simulink library "tllib"  (R2015a)
settings: Solver=ode45  StartTime=0.0  StopTime=10.0  RelTol=1e-3
PostLoadFcn:
  | load_system('simulink')
libraries: simulink x6, tllib x3
(part 1 of 2)
CloseFcn:
  | if (bdIsLoaded('simulink')) && (strcmp(get_param('simulink', 'open'), 'off'))
  | close_system('simulink')
  | end;
settings Model: Creator=dSPACE GmbH  LastModifiedBy=dSPACE GmbH

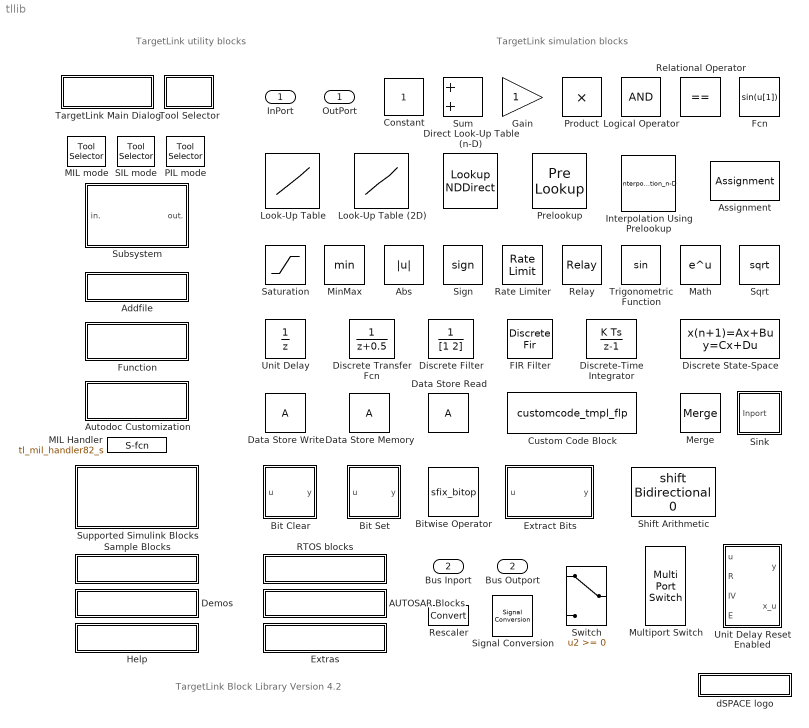
== system tllib ==
  note: TargetLink utility blocks
  note: TargetLink simulation blocks
  note: TargetLink Block Library Version 4.2
  InPort : Inport  mask(TL_Inport){data={'date',730486}}
      settings: CopyFcn=if exist('tl_copyfcntllib', 'file') == 2, tl_copyfcntllib(gcbh); end;  DeleteFcn=if exist('delete_tlblock','file')==2,delete_tlblock(gcbh);end  NameChangeFcn=if exist('rename_tlblock','file')==2,rename_tlblock(gcbh);end  OpenFcn=if exist('tl_open_blockdlg','file')==2,tl_open_blockdlg(gcbh);else,open_system(gcbh,'parameter');end
      mask Help: eval(['if exist(''tl_online_help'',''file'') == 2, tl_online_help(''Topic'',''TL_Inport''),else, web([''jar:file:///'',matlabroot,''/help/toolbox/simulink/help.jar!/slref/' lower(get_param(gcbh,'Blocktype')) '.html''], ''-helpbrowser''),end'])
      mask Display: plot([0.2 0.35 NaN 0.65 0.8],[0 1 NaN 0 1]);
  Bus Inport : Inport  Port=2  mask(TL_BusInport){data={'date',730486}}
      settings: CopyFcn=if exist('tl_copyfcntllib', 'file') == 2, tl_copyfcntllib(gcbh); end;  DeleteFcn=if exist('delete_tlblock','file')==2,delete_tlblock(gcbh);end  NameChangeFcn=if exist('rename_tlblock','file')==2,rename_tlblock(gcbh);end  OpenFcn=if exist('tl_open_blockdlg','file')==2,tl_open_blockdlg(gcbh);else,open_system(gcbh,'parameter');end
      mask Help: eval(['if exist(''tl_online_help'',''file'') == 2, tl_online_help(''Topic'',''TL_Inport''),else, web([''jar:file:///'',matlabroot,''/help/toolbox/simulink/help.jar!/slref/' lower(get_param(gcbh,'Blocktype')) '.html''], ''-helpbrowser''),end'])
      mask Display: plot([0.2 0.35 NaN 0.65 0.8],[0 1 NaN 0 1]);
  AUTOSAR Blocks : Subsystem
      settings: OpenFcn=tl_openfcntllib('tl_autosar_lib');
      mask Display: disp('AUTOSAR blocks')
  Abs : Abs  mask(TL_Abs){data={'date',730486}}
      settings: CopyFcn=if exist('tl_copyfcntllib', 'file') == 2, tl_copyfcntllib(gcbh); end;  DeleteFcn=if exist('delete_tlblock','file')==2,delete_tlblock(gcbh);end  NameChangeFcn=if exist('rename_tlblock','file')==2,rename_tlblock(gcbh);end  OpenFcn=if exist('tl_open_blockdlg','file')==2,tl_open_blockdlg(gcbh);else,open_system(gcbh,'parameter');end
      mask Help: eval(['if exist(''tl_online_help'',''file'') == 2, tl_online_help(''Topic'',''TL_Abs''),else, web([''jar:file:///'',matlabroot,''/help/toolbox/simulink/help.jar!/slref/' lower(get_param(gcbh,'Blocktype')) '.html''], ''-helpbrowser''),end'])
      mask Display: plot([-0.1, 1.05, NaN, -0.1, 1.05],[.01, .01, NaN, .99, .99]);
  Addfile : Subsystem  mask(TL_AddFile){data={'date',730486}, displayString=Link "untitled.c"}
      mask help: TargetLink Addfile block: It is used to add user-supplied source code files to the generated production code application. In full-featured mode it provides a graphical user interface.
      mask init:
      | if exist('tlOperationMode','file')==2
      |    if strcmp(tlOperationMode('get'),'full-featured')
      |       set_param(gcbh,'BackgroundColor','green');
      |    else
      |       set_param(gcbh,'BackgroundColor','[0.6,0.6,0.6]');
      |    end
      | else
      |    set_param(gcbh,'BackgroundColor','[0.6,0.6,0.6]');
      | end
      settings: DeleteFcn=if exist('delete_tlblock','file')==2,delete_tlblock(gcbh);end  NameChangeFcn=if exist('rename_tlblock','file')==2,rename_tlblock(gcbh);end  OpenFcn=if exist('tl_open_blockdlg','file')==2,tl_open_blockdlg(gcbh);else,open_system(gcbh,'mask');end
      mask Help: eval('if exist(''tl_online_help'',''file'') == 2, tl_online_help(''Topic'',get_param(gcbh,''MaskType'')),end')
      mask Display: disp(displayString);
  Assignment : Assignment  mask(TL_Assignment){data={'date',730486}}
      settings: CopyFcn=if exist('tl_copyfcntllib', 'file') == 2, tl_copyfcntllib(gcbh); end;  DeleteFcn=if exist('delete_tlblock','file')==2,delete_tlblock(gcbh);end  NameChangeFcn=if exist('rename_tlblock','file')==2,rename_tlblock(gcbh);end  OpenFcn=if exist('tl_open_blockdlg','file')==2,tl_open_blockdlg(gcbh);else,open_system(gcbh,'parameter');end
      mask Help: eval(['if exist(''tl_online_help'',''file'') == 2, tl_online_help(''Topic'',''TL_Assignment''),else, web([''jar:file:///'',matlabroot,''/help/toolbox/simulink/help.jar!/slref/' lower(get_param(gcbh,'Blocktype')) '.html''], ''-helpbrowser''),end'])
      mask Display: plot([-0.1, 1.05, NaN, -0.1, 1.05],[.01, .01, NaN, .99, .99]);
  Autodoc Customization : Subsystem  mask(TL_Autodoc){data={'date',730486}, displayString=|}
      mask displayString=|
      | Autodoc
      | Customization
      mask help: TargetLink Autodoc Customization block: It is designed for use with TargetLink Document Generation Tool. It can be placed anywhere in Model and allows inserting of user comments or/and screen shots into generated documentation.
      settings: DeleteFcn=if exist('delete_tlblock','file')==2,delete_tlblock(gcbh);end  NameChangeFcn=if exist('rename_tlblock','file')==2,rename_tlblock(gcbh);end  OpenFcn=if exist('tl_open_blockdlg','file')==2,tl_open_blockdlg(gcbh);else,open_system(gcbh,'mask');end
      mask Help: eval('if exist(''tl_online_help'',''file'') == 2, tl_online_help(''Topic'',get_param(gcbh,''MaskType'')),end')
      mask Display: disp(displayString);
  Bit Clear : Subsystem  mask(TL_BitClear){iBit=0, data={'date',730486}}
      mask prompts: iBit "Simulink:masks:IndexOfBit0IsLeastSignificant_MP"
      mask help: Simulink:masks:BitClear_MD
      mask init:
      | if length(iBit) == 1
      |   dispStr = sprintf('Clear\nbit %d',double(iBit));
      | else
      |   dispStr=sprintf('Vector\nBit Clear');
      | end
      settings: DeleteFcn=if exist('delete_tlblock','file')==2,delete_tlblock(gcbh);end  NameChangeFcn=if exist('rename_tlblock','file')==2,rename_tlblock(gcbh);end  OpenFcn=if exist('tl_open_blockdlg','file')==2,tl_open_blockdlg(gcbh);else,open_system(gcbh,'mask');end
      mask Help: eval(['if exist(''tl_online_help'',''file'') == 2, tl_online_help(''Topic'',''TL_BitClear''),else, web([''jar:file:///'',matlabroot,''/help/toolbox/simulink/help.jar!/slref/bitclear.html''], ''-helpbrowser''),end'])
      mask Display:
      | disp(dispStr)
      | plot([-0.1, 1.05, NaN, -0.1, 1.05],[.01, .01, NaN, .99, .99]);
  Bit Set : Subsystem  mask(TL_BitSet){iBit=0, data={'date',730486}}
      mask prompts: iBit "Simulink:masks:IndexOfBit0IsLeastSignificant_MP"
      mask help: Simulink:masks:BitSet_MD
      mask init:
      | if length(iBit) == 1
      |   dispStr = sprintf('Set\nbit %d',double(iBit));
      | else
      |   dispStr=sprintf('Vector\nBit Set');
      | end
      settings: DeleteFcn=if exist('delete_tlblock','file')==2,delete_tlblock(gcbh);end  NameChangeFcn=if exist('rename_tlblock','file')==2,rename_tlblock(gcbh);end  OpenFcn=if exist('tl_open_blockdlg','file')==2,tl_open_blockdlg(gcbh);else,open_system(gcbh,'mask');end
      mask Help: eval(['if exist(''tl_online_help'',''file'') == 2, tl_online_help(''Topic'',''TL_BitSet''),else, web([''jar:file:///'',matlabroot,''/help/toolbox/simulink/help.jar!/slref/bitset.html''], ''-helpbrowser''),end'])
      mask Display:
      | disp(dispStr)
      | plot([-0.1, 1.05, NaN, -0.1, 1.05],[.01, .01, NaN, .99, .99]);
  Bitwise Operator : S-Function  FunctionName=sfix_bitop  Parameters=UseBitMask,NumInputPorts,BitMask,BitMaskRealWorld,logicop  mask(TL_BitwiseOperator){logicop=AND, UseBitMask=on, NumInputPorts=1, BitMask=bin2dec('11011001'), BitMaskRealWorld=Stored Integer, data={'date',730486}}
      mask prompts: logicop "Simulink:masks:Operator_MP"; UseBitMask "Simulink:masks:UseBitMask_MP"; NumInputPorts "Simulink:masks:NumberOfInputPorts_MP"; BitMask "Simulink:masks:BitMask_MP"; BitMaskRealWorld "Simulink:masks:TreatMaskAs_MP"
      mask help: Simulink:masks:BitwiseOperator_MD
      mask init:
      | str = '';
      | if UseBitMask
      |   [m,n] = size(BitMask);
      |   if ischar(BitMask)
      |     len = m;
      |     n = 1;
      |   else
      |     len = m * n;
      |   end
      |   internalBitMask = zeros(m,n);
      |   if isnumeric(BitMask)
      |     if ~isreal(BitMask)
      |       error(DAStudio.message('Simulink:blocks:BitMaskNotComplex'));
      |     end
      |     for i=1:len,
      |       internalBitMask(i) = BitMask(i);
      |     end
      |   elseif ischar(BitMask)
      |     for i=1:m,
      |       internalBitMask(i) = hex2dec(BitMask(i,:));
      |     end
      |   elseif iscell(BitMask)
      |     for i=1:len,
      |       if isnumeric( BitMask{i} )
      |         internalBitMask(i) = BitMask{i};
      |       elseif ischar( BitMask{i} )
      |         internalBitMask(i) = hex2dec(BitMask{i});
      |       else
      |         errordlg(['Data type is not supported at cell item ', num2str(i) ]);
      |       end
      |     end
      |   end
      |   BitMask = internalBitMask;
      |   for i=1:len
      |     if BitMask(i) > (2^52)-1
      |       error(DAStudio.message('Simulink:blocks:BitMaskWordLengthTooLarge')); 
      |     end
      |   end 
      |   if len == 1
      |      if BitMaskRealWorld == 1 || BitMask(1) < 0
      |        str=num2str(BitMask(1));
      |      else
      |        str=['0x',dec2hex(floor(BitMask(1)))];
      |      end
      |   else
      |      str='Masks';
      |   end
      | else
      |   BitMask = 0;
      |   str='';
      | end
      settings: DeleteFcn=if exist('delete_tlblock','file')==2,delete_tlblock(gcbh);end  NameChangeFcn=if exist('rename_tlblock','file')==2,rename_tlblock(gcbh);end  OpenFcn=if exist('tl_open_blockdlg','file')==2,tl_open_blockdlg(gcbh);else,open_system(gcbh,'mask');end
      mask Help: eval(['if exist(''tl_online_help'',''file'') == 2, tl_online_help(''Topic'',''TL_BitwiseOperator''),else, web([''jar:file:///'',matlabroot,''/help/toolbox/simulink/help.jar!/slref/bitwiseoperator.html''], ''-helpbrowser''),end'])
      mask TypeOptions logicop: Simulink:masks:AND | Simulink:masks:OR | Simulink:masks:NAND | Simulink:masks:NOR | Simulink:masks:XOR | Simulink:masks:NOT
      mask Callback logicop: tl_handle_bitwiseblock(gcbh)
      mask Callback UseBitMask: tl_handle_bitwiseblock(gcbh)
      mask TypeOptions BitMaskRealWorld: Simulink:masks:RealWorldValue | Simulink:masks:StoredInteger
      mask Display:
      | fprintf(['Bitwise\n',logicop,'\n',str])
      | plot([-0.1, 1.05, NaN, -0.1, 1.05],[.01, .01, NaN, .99, .99]);
  Constant : Constant  mask(TL_Constant){data={'date',730486}}
      settings: CopyFcn=if exist('tl_copyfcntllib', 'file') == 2, tl_copyfcntllib(gcbh); end;  DeleteFcn=if exist('delete_tlblock','file')==2,delete_tlblock(gcbh);end  NameChangeFcn=if exist('rename_tlblock','file')==2,rename_tlblock(gcbh);end  OpenFcn=if exist('tl_open_blockdlg','file')==2,tl_open_blockdlg(gcbh);else,open_system(gcbh,'parameter');end
      mask Help: eval(['if exist(''tl_online_help'',''file'') == 2, tl_online_help(''Topic'',''TL_Constant''),else, web([''jar:file:///'',matlabroot,''/help/toolbox/simulink/help.jar!/slref/' lower(get_param(gcbh,'Blocktype')) '.html''], ''-helpbrowser''),end'])
      mask Display: plot([-0.1, 1.05, NaN, -0.1, 1.05],[.01, .01, NaN, .99, .99]);
  Custom Code Block : S-Function  FunctionName=customcode_tmpl_flp  Parameters=dt,x01,p  mask(TL_CustomCode){data={'date',730486}, dt=-1, x01=0, p=0}
      mask help:
      | TargetLink Custom Code block:
      | Allows to insert custom code into a TargetLink application.
      settings: CopyFcn=if exist('tl_copyfcntllib', 'file') == 2, tl_copyfcntllib(gcbh); end;  DeleteFcn=if exist('delete_tlblock','file')==2,delete_tlblock(gcbh);end  NameChangeFcn=if exist('rename_tlblock','file')==2,rename_tlblock(gcbh);end  OpenFcn=if exist('tl_open_blockdlg','file')==2,tl_open_blockdlg(gcbh);else,open_system(gcbh,'parameter');end
      mask Help: eval('if exist(''tl_online_help'',''file'') == 2, tl_online_help(''Topic'',get_param(gcbh,''MaskType'')),end')
      mask Display:
      | plot([-0.1, 1.05, NaN, -0.1, 1.05],[.01, .01, NaN, .99, .99]);
      | ; disp('customcode_tmpl.c');port_label('input',1,'u');port_label('output',1,'y');
  Data Store Memory : DataStoreMemory  ReadBeforeWriteMsg=warning  WriteAfterWriteMsg=warning  WriteAfterReadMsg=warning  mask(TL_DataStoreMemory){data={'date',730486}}
      settings: CopyFcn=if exist('tl_copyfcntllib', 'file') == 2, tl_copyfcntllib(gcbh); end;  DeleteFcn=if exist('delete_tlblock','file')==2,delete_tlblock(gcbh);end  NameChangeFcn=if exist('rename_tlblock','file')==2,rename_tlblock(gcbh);end  OpenFcn=if exist('tl_open_blockdlg','file')==2,tl_open_blockdlg(gcbh);else,open_system(gcbh,'parameter');end
      mask Help: eval(['if exist(''tl_online_help'',''file'') == 2, tl_online_help(''Topic'',''TL_DataStoreMemory''),else, web([''jar:file:///'',matlabroot,''/help/toolbox/simulink/help.jar!/slref/' lower(get_param(gcbh,'Blocktype')) '.html''], ''-helpbrowser''),end'])
      mask Display:
      | plot([-0.1, 1.05, NaN, -0.1, 1.05],[.01, .01, NaN, .99, .99]);
      | plot([-0.1, 1.05, NaN, -0.1, 1.05],[.01, .01, NaN, .99, .99]);
  Data Store Read : DataStoreRead  mask(TL_DataStoreRead){data={'date',730486}}
      settings: CopyFcn=if exist('tl_copyfcntllib', 'file') == 2, tl_copyfcntllib(gcbh); end;  DeleteFcn=if exist('delete_tlblock','file')==2,delete_tlblock(gcbh);end  NameChangeFcn=if exist('rename_tlblock','file')==2,rename_tlblock(gcbh);end  OpenFcn=if exist('tl_open_blockdlg','file')==2,tl_open_blockdlg(gcbh);else,open_system(gcbh,'parameter');end
      mask Help: eval(['if exist(''tl_online_help'',''file'') == 2, tl_online_help(''Topic'',''TL_DataStoreRead''),else, web([''jar:file:///'',matlabroot,''/help/toolbox/simulink/help.jar!/slref/' lower(get_param(gcbh,'Blocktype')) '.html''], ''-helpbrowser''),end'])
      mask Display:
      | plot([-0.1, 1.05, NaN, -0.1, 1.05],[.01, .01, NaN, .99, .99]);
      | plot([-0.1, 1.05, NaN, -0.1, 1.05],[.01, .01, NaN, .99, .99]);
  Data Store Write : DataStoreWrite  mask(TL_DataStoreWrite){data={'date',730486}}
      settings: CopyFcn=if exist('tl_copyfcntllib', 'file') == 2, tl_copyfcntllib(gcbh); end;  DeleteFcn=if exist('delete_tlblock','file')==2,delete_tlblock(gcbh);end  NameChangeFcn=if exist('rename_tlblock','file')==2,rename_tlblock(gcbh);end  OpenFcn=if exist('tl_open_blockdlg','file')==2,tl_open_blockdlg(gcbh);else,open_system(gcbh,'parameter');end
      mask Help: eval(['if exist(''tl_online_help'',''file'') == 2, tl_online_help(''Topic'',''TL_DataStoreWrite''),else, web([''jar:file:///'',matlabroot,''/help/toolbox/simulink/help.jar!/slref/' lower(get_param(gcbh,'Blocktype')) '.html''], ''-helpbrowser''),end'])
      mask Display:
      | plot([-0.1, 1.05, NaN, -0.1, 1.05],[.01, .01, NaN, .99, .99]);
      | plot([-0.1, 1.05, NaN, -0.1, 1.05],[.01, .01, NaN, .99, .99]);
  Demos : Subsystem
      settings: OpenFcn=tl_demos
      mask Display: disp('Demos')
  Direct Look-Up Table (n-D) : LookupNDDirect  Table=[4 5 6; 16 19 20; 10 18 23]  mask(TL_LookupNDDirect){data={'date',730486}}
      settings: CopyFcn=if exist('tl_copyfcntllib', 'file') == 2, tl_copyfcntllib(gcbh); end;  DeleteFcn=if exist('delete_tlblock','file')==2,delete_tlblock(gcbh);end  NameChangeFcn=if exist('rename_tlblock','file')==2,rename_tlblock(gcbh);end  OpenFcn=if exist('tl_open_blockdlg','file')==2,tl_open_blockdlg(gcbh);else,open_system(gcbh,'parameter');end
      mask Help: eval(['if exist(''tl_online_help'',''file'') == 2, tl_online_help(''Topic'',''TL_LookupNDDirect''),else, web([''jar:file:///'',matlabroot,''/help/toolbox/simulink/help.jar!/slref/directlookuptablend.html''], ''-helpbrowser''),end'])
      mask Display: plot([-0.1, 1.05, NaN, -0.1, 1.05],[.01, .01, NaN, .99, .99]);
  Discrete Transfer Fcn : DiscreteTransferFcn  Numerator=1  mask(TL_DiscreteTransferFcn){data={'date',730486}}
      settings: CopyFcn=if exist('tl_copyfcntllib', 'file') == 2, tl_copyfcntllib(gcbh); end;  DeleteFcn=if exist('delete_tlblock','file')==2,delete_tlblock(gcbh);end  NameChangeFcn=if exist('rename_tlblock','file')==2,rename_tlblock(gcbh);end  OpenFcn=if exist('tl_open_blockdlg','file')==2,tl_open_blockdlg(gcbh);else,open_system(gcbh,'parameter');end
      mask Help: eval(['if exist(''tl_online_help'',''file'') == 2, tl_online_help(''Topic'',''TL_DiscreteTransferFcn''),else, web([''jar:file:///'',matlabroot,''/help/toolbox/simulink/help.jar!/slref/' lower(get_param(gcbh,'Blocktype')) '.html''], ''-helpbrowser''),end'])
      mask Display: plot([-0.1, 1.05, NaN, -0.1, 1.05],[.01, .01, NaN, .99, .99]);
  Discrete Filter : DiscreteFilter  Numerator=1  Denominator=[1 2]  mask(TL_DiscreteFilter){data={'date',730486}}
      settings: CopyFcn=if exist('tl_copyfcntllib', 'file') == 2, tl_copyfcntllib(gcbh); end;  DeleteFcn=if exist('delete_tlblock','file')==2,delete_tlblock(gcbh);end  NameChangeFcn=if exist('rename_tlblock','file')==2,rename_tlblock(gcbh);end  OpenFcn=if exist('tl_open_blockdlg','file')==2,tl_open_blockdlg(gcbh);else,open_system(gcbh,'parameter');end
      mask Help: eval(['if exist(''tl_online_help'',''file'') == 2, tl_online_help(''Topic'',''TL_DiscreteFilter''),else, web([''jar:file:///'',matlabroot,''/help/toolbox/simulink/help.jar!/slref/' lower(get_param(gcbh,'Blocktype')) '.html''], ''-helpbrowser''),end'])
      mask Display: plot([-0.1, 1.05, NaN, -0.1, 1.05],[.01, .01, NaN, .99, .99]);
  Discrete State-Space : DiscreteStateSpace  SampleTime=-1  mask(TL_DiscreteStateSpace){data={'date',730486}}
      settings: CopyFcn=if exist('tl_copyfcntllib', 'file') == 2, tl_copyfcntllib(gcbh); end;  DeleteFcn=if exist('delete_tlblock','file')==2,delete_tlblock(gcbh);end  NameChangeFcn=if exist('rename_tlblock','file')==2,rename_tlblock(gcbh);end  OpenFcn=if exist('tl_open_blockdlg','file')==2,tl_open_blockdlg(gcbh);else,open_system(gcbh,'parameter');end
      mask Help: eval(['if exist(''tl_online_help'',''file'') == 2, tl_online_help(''Topic'',''TL_DiscreteStateSpace''),else, web([''jar:file:///'',matlabroot,''/help/toolbox/simulink/help.jar!/slref/' lower(get_param(gcbh,'Blocktype')) '.html''], ''-helpbrowser''),end'])
      mask Display: plot([-0.1, 1.05, NaN, -0.1, 1.05],[.01, .01, NaN, .99, .99]);
  Discrete-Time Integrator : DiscreteIntegrator  SampleTime=-1  mask(TL_DiscreteIntegrator){data={'date',730486}}
      settings: CopyFcn=if exist('tl_copyfcntllib', 'file') == 2, tl_copyfcntllib(gcbh); end;  DeleteFcn=if exist('delete_tlblock','file')==2,delete_tlblock(gcbh);end  NameChangeFcn=if exist('rename_tlblock','file')==2,rename_tlblock(gcbh);end  OpenFcn=if exist('tl_open_blockdlg','file')==2,tl_open_blockdlg(gcbh);else,open_system(gcbh,'parameter');end
      mask Help: eval(['if exist(''tl_online_help'',''file'') == 2, tl_online_help(''Topic'',''TL_DiscreteIntegrator''),else, web([''jar:file:///'',matlabroot,''/help/toolbox/simulink/help.jar!/slref/' lower(get_param(gcbh,'Blocktype')) '.html''], ''-helpbrowser''),end'])
      mask Display: plot([-0.1, 1.05, NaN, -0.1, 1.05],[.01, .01, NaN, .99, .99]);
  Extract Bits : Subsystem  mask(TL_ExtractBits){bitsToExtract=Upper half, numBits=8, bitIdxRange=[0 7], outScalingMode=Treat bit field as an integer, data={'date',730486}}
      mask prompts: bitsToExtract "Simulink:masks:BitsToExtract_MP"; numBits "Simulink:masks:NumberOfBits_MP"; bitIdxRange "Simulink:masks:BitIndicesstartEnd0basedRelativeToLSB_MP"; outScalingMode "Simulink:masks:OutputScalingMode_MP"
      mask help: Simulink:masks:ExtractBits_MD
      mask init:
      | if get_param(0, 'version') < 7.1
      |     str = fixpt_extractbits_mask('icon');
      | else
      |     str = fixpt_extractbits_mask('icon', numBits, bitIdxRange);
      | end
      | fixpt_extractbits_mask_script;
      settings: CopyFcn=if exist('tl_reset_reviewflag') == 2, tl_reset_reviewflag(gcbh); end;  DeleteFcn=if exist('delete_tlblock','file')==2,delete_tlblock(gcbh);end  NameChangeFcn=if exist('rename_tlblock','file')==2,rename_tlblock(gcbh);end  OpenFcn=if exist('tl_open_blockdlg','file')==2,tl_open_blockdlg(gcbh);else,open_system(gcbh,'mask');end
      mask Help: eval(['if exist(''tl_online_help'',''file'') == 2, tl_online_help(''Topic'',''TL_ExtractBits''),else, web([''jar:file:///'',matlabroot,''/help/toolbox/simulink/help.jar!/slref/extractbits.html''], ''-helpbrowser''),end'])
      mask TypeOptions bitsToExtract: Simulink:masks:UpperHalf | Simulink:masks:LowerHalf | Simulink:masks:RangeStartingWithMostSignificantBit | Simulink:masks:RangeEndingWithLeastSignificantBit | Simulink:masks:RangeOfBits
      mask Callback bitsToExtract: fixpt_extractbits_mask;
      mask TypeOptions outScalingMode: Simulink:masks:PreserveFixedPointScaling | Simulink:masks:TreatBitFieldAsAnInteger
      mask Display:
      | disp(str);
      | plot([-0.1, 1.05, NaN, -0.1, 1.05],[.01, .01, NaN, .99, .99]);
  Extras : Subsystem
      settings: CopyFcn=set_param(gcbh,'ReferenceBlock','');
      mask Display: disp('Extras')
  FIR Filter : DiscreteFir  Coefficients="[0.0338    0.2401    0.4521    0.2401    0.0338]"  mask(TL_FIRFilter){data={'date',730486}}
      settings: CopyFcn=if exist('tl_copyfcntllib', 'file') == 2, tl_copyfcntllib(gcbh); end;  DeleteFcn=if exist('delete_tlblock','file')==2,delete_tlblock(gcbh);end  NameChangeFcn=if exist('rename_tlblock','file')==2,rename_tlblock(gcbh);end  OpenFcn=if exist('tl_open_blockdlg','file')==2,tl_open_blockdlg(gcbh);else,open_system(gcbh,'parameter');end
      mask Help: eval(['if exist(''tl_online_help'',''file'') == 2, tl_online_help(''Topic'',''TL_FIRFilter''),else, web([''jar:file:///'',matlabroot,''/help/toolbox/simulink/help.jar!/slref/' lower(get_param(gcbh,'Blocktype')) '.html''], ''-helpbrowser''),end'])
      mask Display: plot([-0.1, 1.05, NaN, -0.1, 1.05],[.01, .01, NaN, .99, .99]);
  Fcn : Fcn  mask(TL_Fcn){data={'date',730486}}
      settings: CopyFcn=if exist('tl_copyfcntllib', 'file') == 2, tl_copyfcntllib(gcbh); end;  DeleteFcn=if exist('delete_tlblock','file')==2,delete_tlblock(gcbh);end  NameChangeFcn=if exist('rename_tlblock','file')==2,rename_tlblock(gcbh);end  OpenFcn=if exist('tl_open_blockdlg','file')==2,tl_open_blockdlg(gcbh);else,open_system(gcbh,'parameter');end
      mask Help: eval(['if exist(''tl_online_help'',''file'') == 2, tl_online_help(''Topic'',''TL_Fcn''),else, web([''jar:file:///'',matlabroot,''/help/toolbox/simulink/help.jar!/slref/' lower(get_param(gcbh,'Blocktype')) '.html''], ''-helpbrowser''),end'])
      mask Display: plot([-0.1, 1.05, NaN, -0.1, 1.05],[.01, .01, NaN, .99, .99]);
  Function : Subsystem  LoadFcn=if exist('tl_loadfcn','file')==2,tl_loadfcn(gcbh);end  mask(TL_Function){data={'date',730486}, displayString=FUNCTION}
      mask help: TargetLink Function block: It is used to generate code for a subsystem in a separate C function. In full-featured mode it provides an graphical user interface.
      mask init:
      | hBlock = gcbh;
      | if exist('tlOperationMode','file')==2
      |    if strcmp(tlOperationMode('get'),'full-featured')
      |       set_param(hBlock,'BackgroundColor','green');
      |    else
      |       set_param(hBlock,'BackgroundColor','[0.6,0.6,0.6]');
      |    end
      | else
      |    set_param(hBlock,'BackgroundColor','[0.6,0.6,0.6]');
      | end
      |  
      | if exist('tl_add_swcparameter','file')==2
      |     tl_add_swcparameter(hBlock);
      | end
      settings: DeleteFcn=if exist('delete_tlblock','file')==2,delete_tlblock(gcbh);end  NameChangeFcn=if exist('rename_tlblock','file')==2,rename_tlblock(gcbh);end  OpenFcn=if exist('tl_open_blockdlg','file')==2,tl_open_blockdlg(gcbh);else,open_system(gcbh,'mask');end
      mask Help: eval('if exist(''tl_online_help'',''file'') == 2, tl_online_help(''Topic'',get_param(gcbh,''MaskType'')),end')
      mask Display: disp(displayString);
  Gain : Gain  mask(TL_Gain){data={'date',730486}}
      settings: CopyFcn=if exist('tl_copyfcntllib', 'file') == 2, tl_copyfcntllib(gcbh); end;  DeleteFcn=if exist('delete_tlblock','file')==2,delete_tlblock(gcbh);end  NameChangeFcn=if exist('rename_tlblock','file')==2,rename_tlblock(gcbh);end  OpenFcn=if exist('tl_open_blockdlg','file')==2,tl_open_blockdlg(gcbh);else,open_system(gcbh,'parameter');end
      mask Help: eval(['if exist(''tl_online_help'',''file'') == 2, tl_online_help(''Topic'',''TL_Gain''),else, web([''jar:file:///'',matlabroot,''/help/toolbox/simulink/help.jar!/slref/' lower(get_param(gcbh,'Blocktype')) '.html''], ''-helpbrowser''),end'])
      mask Display: plot([0, .88, 0],[.05, .5, .93]);
  Help : Subsystem
      settings: OpenFcn=ds_open_help('tllib');
      mask Display: disp('Help')
  Interpolation Using Prelookup : Interpolation_n-D  Table=sqrt([1:10]'*[1:10])  ExtrapMethod=Clip  ValidIndexMayReachLast=on  mask(TL_Interpolation_n-D){data={'date',730486}}
      settings: CopyFcn=if exist('tl_copyfcntllib', 'file') == 2, tl_copyfcntllib(gcbh); end;  DeleteFcn=if exist('delete_tlblock','file')==2,delete_tlblock(gcbh);end  NameChangeFcn=if exist('rename_tlblock','file')==2,rename_tlblock(gcbh);end  OpenFcn=if exist('tl_open_blockdlg','file')==2,tl_open_blockdlg(gcbh);else,open_system(gcbh,'parameter');end
      mask Help: eval(['if exist(''tl_online_help'',''file'') == 2, tl_online_help(''Topic'',''TL_Interpolation_n-D''),else, web([''jar:file:///'',matlabroot,''/help/toolbox/simulink/help.jar!/slref/' lower(get_param(gcbh,'Blocktype')) '.html''], ''-helpbrowser''),end'])
      mask Display: plot([-0.1, 1.05, NaN, -0.1, 1.05],[.01, .01, NaN, .99, .99]);
  Logical Operator : Logic  AllPortsSameDT=off  OutDataTypeStr=boolean  mask(TL_LogicalOperator){data={'date',730486}}
      settings: CopyFcn=if exist('tl_copyfcntllib', 'file') == 2, tl_copyfcntllib(gcbh); end;  DeleteFcn=if exist('delete_tlblock','file')==2,delete_tlblock(gcbh);end  NameChangeFcn=if exist('rename_tlblock','file')==2,rename_tlblock(gcbh);end  OpenFcn=if exist('tl_open_blockdlg','file')==2,tl_open_blockdlg(gcbh);else,open_system(gcbh,'parameter');end
      mask Help: eval(['if exist(''tl_online_help'',''file'') == 2, tl_online_help(''Topic'',''TL_LogicalOperator''),else, web([''jar:file:///'',matlabroot,''/help/toolbox/simulink/help.jar!/slref/' lower(get_param(gcbh,'Blocktype')) '.html''], ''-helpbrowser''),end'])
      mask Display: plot([-0.1, 1.05, NaN, -0.1, 1.05],[.01, .01, NaN, .99, .99]);
  Look-Up Table : Lookup_n-D  NumberOfTableDimensions=1  BreakpointsForDimension1=[-5:5]  BreakpointsForDimension2=[1:3]  IndexSearchMethod=Linear search  Table=tanh([-5:5])  ExtrapMethod=Clip  InternalRulePriority=Speed  RndMeth=Simplest  InputSameDT=on  mask(TL_Lookup1D){data={'date',730486}}
      settings: CopyFcn=if exist('tl_copyfcntllib', 'file') == 2, tl_copyfcntllib(gcbh); end;  DeleteFcn=if exist('delete_tlblock','file')==2,delete_tlblock(gcbh);end  NameChangeFcn=if exist('rename_tlblock','file')==2,rename_tlblock(gcbh);end  OpenFcn=if exist('tl_open_blockdlg','file')==2,tl_open_blockdlg(gcbh);else,open_system(gcbh,'parameter');end
      mask Help: eval(['if exist(''tl_online_help'',''file'') == 2, tl_online_help(''Topic'',''TL_Lookup1D''),else, web([''jar:file:///'',matlabroot,''/help/toolbox/simulink/help.jar!/slref/' lower(get_param(gcbh,'Blocktype')) '.html''], ''-helpbrowser''),end'])
      mask Display: plot([-0.1, 1.05, NaN, -0.1, 1.05],[.01, .01, NaN, .99, .99]);
  Look-Up Table (2D) : Lookup_n-D  BreakpointsForDimension1=[1:3]  BreakpointsForDimension2=[1:3]  IndexSearchMethod=Linear search  ExtrapMethod=Clip  InternalRulePriority=Speed  RndMeth=Simplest  InputSameDT=on  mask(TL_Lookup2D){data={'date',730486}}
      settings: CopyFcn=if exist('tl_copyfcntllib', 'file') == 2, tl_copyfcntllib(gcbh); end;  DeleteFcn=if exist('delete_tlblock','file')==2,delete_tlblock(gcbh);end  NameChangeFcn=if exist('rename_tlblock','file')==2,rename_tlblock(gcbh);end  OpenFcn=if exist('tl_open_blockdlg','file')==2,tl_open_blockdlg(gcbh);else,open_system(gcbh,'parameter');end
      mask Help: eval(['if exist(''tl_online_help'',''file'') == 2, tl_online_help(''Topic'',''TL_Lookup2D''),else, web([''jar:file:///'',matlabroot,''/help/toolbox/simulink/help.jar!/slref/' lower(get_param(gcbh,'Blocktype')) '.html''], ''-helpbrowser''),end'])
      mask Display: plot([-0.1, 1.05, NaN, -0.1, 1.05],[.01, .01, NaN, .99, .99]);
  MIL Handler : S-Function  FunctionName=tl_mil_handler82_s  mask(TL_MilHandler){data={'date',730486}}
      mask help: TargetLink MIL Handler
      mask init:
      | if get_param(0,'version') <= 8.2
      |     fname = sprintf('tl_mil_handler%d_s', 10*get_param(0,'Version'));
      | else
      | fname = sprintf('tl_mil_handler82_s');
      | end
      | set_param(gcbh,'FunctionName', fname, 'SFunctionModules','''''');
      settings: CopyFcn=if exist('tl_copyfcn') == 2, tl_copyfcn(gcbh); end  DeleteFcn=if exist('delete_tlblock','file')==2,delete_tlblock(gcbh);end  NameChangeFcn=if exist('rename_tlblock','file')==2,rename_tlblock(gcbh);end  OpenFcn=open_system(gcbh,'mask')
      mask Help: eval('if exist(''tl_online_help'',''file'') == 2, tl_online_help(''Topic'',get_param(gcbh,''MaskType'')),end')
      mask Display: disp('MIL Handler')
  MIL mode : tllib/Tool Selector  Description=MIL\nmode  data={'date',730486}
  Math : Math  SaturateOnIntegerOverflow=on  mask(TL_Math){data={'date',730486}}
      settings: CopyFcn=if exist('tl_copyfcntllib', 'file') == 2, tl_copyfcntllib(gcbh); end;  DeleteFcn=if exist('delete_tlblock','file')==2,delete_tlblock(gcbh);end  NameChangeFcn=if exist('rename_tlblock','file')==2,rename_tlblock(gcbh);end  OpenFcn=if exist('tl_open_blockdlg','file')==2,tl_open_blockdlg(gcbh);else,open_system(gcbh,'parameter');end
      mask Help: eval(['if exist(''tl_online_help'',''file'') == 2, tl_online_help(''Topic'',''TL_Math''),else, web([''jar:file:///'',matlabroot,''/help/toolbox/simulink/help.jar!/slref/' lower(get_param(gcbh,'Blocktype')) '.html''], ''-helpbrowser''),end'])
      mask Display: plot([-0.1, 1.05, NaN, -0.1, 1.05],[.01, .01, NaN, .99, .99]);
  Merge : Merge  mask(TL_Merge){data={'date',730486}}
      settings: CopyFcn=if exist('tl_copyfcntllib', 'file') == 2, tl_copyfcntllib(gcbh); end;  DeleteFcn=if exist('delete_tlblock','file')==2,delete_tlblock(gcbh);end  NameChangeFcn=if exist('rename_tlblock','file')==2,rename_tlblock(gcbh);end  OpenFcn=if exist('tl_open_blockdlg','file')==2,tl_open_blockdlg(gcbh);else,open_system(gcbh,'parameter');end
      mask Help: eval(['if exist(''tl_online_help'',''file'') == 2, tl_online_help(''Topic'',''TL_Merge''),else, web([''jar:file:///'',matlabroot,''/help/toolbox/simulink/help.jar!/slref/' lower(get_param(gcbh,'Blocktype')) '.html''], ''-helpbrowser''),end'])
      mask Display: plot([-0.1, 1.05, NaN, -0.1, 1.05],[.01, .01, NaN, .99, .99]);
  MinMax : MinMax  Inputs=2  mask(TL_MinMax){data={'date',730486}}
      settings: CopyFcn=if exist('tl_copyfcntllib', 'file') == 2, tl_copyfcntllib(gcbh); end;  DeleteFcn=if exist('delete_tlblock','file')==2,delete_tlblock(gcbh);end  NameChangeFcn=if exist('rename_tlblock','file')==2,rename_tlblock(gcbh);end  OpenFcn=if exist('tl_open_blockdlg','file')==2,tl_open_blockdlg(gcbh);else,open_system(gcbh,'parameter');end
      mask Help: eval(['if exist(''tl_online_help'',''file'') == 2, tl_online_help(''Topic'',''TL_MinMax''),else, web([''jar:file:///'',matlabroot,''/help/toolbox/simulink/help.jar!/slref/' lower(get_param(gcbh,'Blocktype')) '.html''], ''-helpbrowser''),end'])
      mask Display: plot([-0.1, 1.05, NaN, -0.1, 1.05],[.01, .01, NaN, .99, .99]);
  Multiport Switch : MultiPortSwitch  mask(TL_MultiPortSwitch){data={'date',730486}}
      settings: CopyFcn=if exist('tl_copyfcntllib', 'file') == 2, tl_copyfcntllib(gcbh); end;  DeleteFcn=if exist('delete_tlblock','file')==2,delete_tlblock(gcbh);end  NameChangeFcn=if exist('rename_tlblock','file')==2,rename_tlblock(gcbh);end  OpenFcn=if exist('tl_open_blockdlg','file')==2,tl_open_blockdlg(gcbh);else,open_system(gcbh,'parameter');end
      mask Help: eval(['if exist(''tl_online_help'',''file'') == 2, tl_online_help(''Topic'',''TL_MultiPortSwitch''),else, web([''jar:file:///'',matlabroot,''/help/toolbox/simulink/help.jar!/slref/' lower(get_param(gcbh,'Blocktype')) '.html''], ''-helpbrowser''),end'])
      mask Display: plot([-0.1, 1.05, NaN, -0.1, 1.05],[.01, .01, NaN, .99, .99]);
  PIL mode : tllib/Tool Selector  Description=PIL\nmode  data={'date',730486}
  Prelookup : PreLookup  UseLastBreakpoint=on  mask(TL_PreLookup){data={'date',730486}}
      settings: CopyFcn=if exist('tl_copyfcntllib', 'file') == 2, tl_copyfcntllib(gcbh); end;  DeleteFcn=if exist('delete_tlblock','file')==2,delete_tlblock(gcbh);end  NameChangeFcn=if exist('rename_tlblock','file')==2,rename_tlblock(gcbh);end  OpenFcn=if exist('tl_open_blockdlg','file')==2,tl_open_blockdlg(gcbh);else,open_system(gcbh,'parameter');end
      mask Help: eval(['if exist(''tl_online_help'',''file'') == 2, tl_online_help(''Topic'',''TL_PreLookup''),else, web([''jar:file:///'',matlabroot,''/help/toolbox/simulink/help.jar!/slref/' lower(get_param(gcbh,'Blocktype')) '.html''], ''-helpbrowser''),end'])
      mask Display: plot([-0.1, 1.05, NaN, -0.1, 1.05],[.01, .01, NaN, .99, .99]);
  Product : Product  Inputs=**  RndMeth=Zero  mask(TL_Product){data={'date',730486}}
      settings: CopyFcn=if exist('tl_copyfcntllib', 'file') == 2, tl_copyfcntllib(gcbh); end;  DeleteFcn=if exist('delete_tlblock','file')==2,delete_tlblock(gcbh);end  NameChangeFcn=if exist('rename_tlblock','file')==2,rename_tlblock(gcbh);end  OpenFcn=if exist('tl_open_blockdlg','file')==2,tl_open_blockdlg(gcbh);else,open_system(gcbh,'parameter');end
      mask Help: eval(['if exist(''tl_online_help'',''file'') == 2, tl_online_help(''Topic'',''TL_Product''),else, web([''jar:file:///'',matlabroot,''/help/toolbox/simulink/help.jar!/slref/' lower(get_param(gcbh,'Blocktype')) '.html''], ''-helpbrowser''),end'])
      mask Display: plot([-0.1, 1.05, NaN, -0.1, 1.05],[.01, .01, NaN, .99, .99]);
  RTOS blocks : Subsystem
      settings: OpenFcn=tl_openfcntllib('tl_rtos_lib');
      mask Display: disp('RTOS blocks')
  Rate Limiter : RateLimiter  SampleTimeMode=inherited  mask(TL_RateLimiter){data={'date',730486}}
      settings: CopyFcn=if exist('tl_copyfcntllib', 'file') == 2, tl_copyfcntllib(gcbh); end;  DeleteFcn=if exist('delete_tlblock','file')==2,delete_tlblock(gcbh);end  NameChangeFcn=if exist('rename_tlblock','file')==2,rename_tlblock(gcbh);end  OpenFcn=if exist('tl_open_blockdlg','file')==2,tl_open_blockdlg(gcbh);else,open_system(gcbh,'parameter');end
      mask Help: eval(['if exist(''tl_online_help'',''file'') == 2, tl_online_help(''Topic'',''TL_RateLimiter''),else, web([''jar:file:///'',matlabroot,''/help/toolbox/simulink/help.jar!/slref/' lower(get_param(gcbh,'Blocktype')) '.html''], ''-helpbrowser''),end'])
      mask Display: plot([-0.1, 1.05, NaN, -0.1, 1.05],[.01, .01, NaN, .99, .99]);
  Relational Operator : RelationalOperator  Operator===  OutDataTypeStr=boolean  mask(TL_RelationalOperator){data={'date',730486}}
      settings: CopyFcn=if exist('tl_copyfcntllib', 'file') == 2, tl_copyfcntllib(gcbh); end;  DeleteFcn=if exist('delete_tlblock','file')==2,delete_tlblock(gcbh);end  NameChangeFcn=if exist('rename_tlblock','file')==2,rename_tlblock(gcbh);end  OpenFcn=if exist('tl_open_blockdlg','file')==2,tl_open_blockdlg(gcbh);else,open_system(gcbh,'parameter');end
      mask Help: eval(['if exist(''tl_online_help'',''file'') == 2, tl_online_help(''Topic'',''TL_RelationalOperator''),else, web([''jar:file:///'',matlabroot,''/help/toolbox/simulink/help.jar!/slref/' lower(get_param(gcbh,'Blocktype')) '.html''], ''-helpbrowser''),end'])
      mask Display: plot([-0.1, 1.05, NaN, -0.1, 1.05],[.01, .01, NaN, .99, .99]);
  Relay : Relay  OnSwitchValue=1  OffSwitchValue=-1  mask(TL_Relay){data={'date',730486}}
      settings: CopyFcn=if exist('tl_copyfcntllib', 'file') == 2, tl_copyfcntllib(gcbh); end;  DeleteFcn=if exist('delete_tlblock','file')==2,delete_tlblock(gcbh);end  NameChangeFcn=if exist('rename_tlblock','file')==2,rename_tlblock(gcbh);end  OpenFcn=if exist('tl_open_blockdlg','file')==2,tl_open_blockdlg(gcbh);else,open_system(gcbh,'parameter');end
      mask Help: eval(['if exist(''tl_online_help'',''file'') == 2, tl_online_help(''Topic'',''TL_Relay''),else, web([''jar:file:///'',matlabroot,''/help/toolbox/simulink/help.jar!/slref/' lower(get_param(gcbh,'Blocktype')) '.html''], ''-helpbrowser''),end'])
      mask Display: plot([-0.1, 1.05, NaN, -0.1, 1.05],[.01, .01, NaN, .99, .99]);
  Rescaler : DataTypeConversion  mask(TL_Rescaler){data={'date',730486}}
      settings: CopyFcn=if exist('tl_copyfcntllib', 'file') == 2, tl_copyfcntllib(gcbh); end;  DeleteFcn=if exist('delete_tlblock','file')==2,delete_tlblock(gcbh);end  NameChangeFcn=if exist('rename_tlblock','file')==2,rename_tlblock(gcbh);end  OpenFcn=if exist('tl_open_blockdlg','file')==2,tl_open_blockdlg(gcbh);else,open_system(gcbh,'parameter');end
      mask Help: eval(['if exist(''tl_online_help'',''file'') == 2, tl_online_help(''Topic'',''TL_Rescaler''),else, web([''jar:file:///'',matlabroot,''/help/toolbox/simulink/help.jar!/slref/' lower(get_param(gcbh,'Blocktype')) '.html''], ''-helpbrowser''),end'])
      mask Display: plot([-0.1, 1.05, NaN, -0.1, 1.05],[.01, .01, NaN, .99, .99]);
  SIL mode : tllib/Tool Selector  Description=SIL\nmode  data={'date',730486}
  Sample Blocks : Subsystem
      settings: OpenFcn=tl_openfcntllib('tlsamples')
      mask Display: disp('Sample blocks')
  Saturation : Saturate  UpperLimit=1  LowerLimit=-1  mask(TL_Saturate){data={'date',730486}}
      settings: CopyFcn=if exist('tl_copyfcntllib', 'file') == 2, tl_copyfcntllib(gcbh); end;  DeleteFcn=if exist('delete_tlblock','file')==2,delete_tlblock(gcbh);end  NameChangeFcn=if exist('rename_tlblock','file')==2,rename_tlblock(gcbh);end  OpenFcn=if exist('tl_open_blockdlg','file')==2,tl_open_blockdlg(gcbh);else,open_system(gcbh,'parameter');end
      mask Help: eval(['if exist(''tl_online_help'',''file'') == 2, tl_online_help(''Topic'',''TL_Saturate''),else, web([''jar:file:///'',matlabroot,''/help/toolbox/simulink/help.jar!/slref/' lower(get_param(gcbh,'Blocktype')) '.html''], ''-helpbrowser''),end'])
      mask Display: plot([-0.1, 1.05, NaN, -0.1, 1.05],[.01, .01, NaN, .99, .99]);
  Shift Arithmetic : ArithShift  LoadFcn=hBlOcK = gcbh; if strcmp(get_param(hBlOcK, 'LinkStatus'), 'resolved'), set_param(hBlOcK, 'LinkStatus', 'none'); set_param(hBlOcK, 'LoadFcn', ''); end; clear('hBlOcK');  mask(TL_ArithShift){data={'date',730486}}
      settings: CopyFcn=if exist('tl_copyfcntllib', 'file') == 2, tl_copyfcntllib(gcbh); end;  DeleteFcn=if exist('delete_tlblock','file')==2,delete_tlblock(gcbh);end  NameChangeFcn=if exist('rename_tlblock','file')==2,rename_tlblock(gcbh);end  OpenFcn=if exist('tl_open_blockdlg','file')==2,tl_open_blockdlg(gcbh);else,open_system(gcbh,'parameter');end
      mask Help: eval(['if exist(''tl_online_help'',''file'') == 2, tl_online_help(''Topic'',''TL_ArithShift''),else, web([''jar:file:///'',matlabroot,''/help/toolbox/simulink/help.jar!/slref/' lower(get_param(gcbh,'Blocktype')) '.html''], ''-helpbrowser''),end'])
      mask Display: plot([-0.1, 1.05, NaN, -0.1, 1.05],[.01, .01, NaN, .99, .99]);
  Sign : Signum  mask(TL_Signum){data={'date',730486}}
      settings: CopyFcn=if exist('tl_copyfcntllib', 'file') == 2, tl_copyfcntllib(gcbh); end;  DeleteFcn=if exist('delete_tlblock','file')==2,delete_tlblock(gcbh);end  NameChangeFcn=if exist('rename_tlblock','file')==2,rename_tlblock(gcbh);end  OpenFcn=if exist('tl_open_blockdlg','file')==2,tl_open_blockdlg(gcbh);else,open_system(gcbh,'parameter');end
      mask Help: eval(['if exist(''tl_online_help'',''file'') == 2, tl_online_help(''Topic'',''TL_Signum''),else, web([''jar:file:///'',matlabroot,''/help/toolbox/simulink/help.jar!/slref/' lower(get_param(gcbh,'Blocktype')) '.html''], ''-helpbrowser''),end'])
      mask Display: plot([-0.1, 1.05, NaN, -0.1, 1.05],[.01, .01, NaN, .99, .99]);
  Signal Conversion : SignalConversion  mask(TL_SignalConversion){data={'date',730486}}
      settings: CopyFcn=if exist('tl_copyfcntllib', 'file') == 2, tl_copyfcntllib(gcbh); end;  DeleteFcn=if exist('delete_tlblock','file')==2,delete_tlblock(gcbh);end  NameChangeFcn=if exist('rename_tlblock','file')==2,rename_tlblock(gcbh);end  OpenFcn=if exist('tl_open_blockdlg','file')==2,tl_open_blockdlg(gcbh);else,open_system(gcbh,'parameter');end
      mask Help: eval(['if exist(''tl_online_help'',''file'') == 2, tl_online_help(''Topic'',''TL_SignalConversion''),else, web([''jar:file:///'',matlabroot,''/help/toolbox/simulink/help.jar!/slref/' lower(get_param(gcbh,'Blocktype')) '.html''], ''-helpbrowser''),end'])
      mask Display: plot([-0.1, 1.05, NaN, -0.1, 1.05],[.01, .01, NaN, .99, .99]);
  Sink : Subsystem  TreatAsAtomicUnit=on  mask(TL_Sink){data={'date',730486}, dt=-1}
      mask help: TargetLink Sink block: It is used to log and display the input vector of arbitrary width during simulation. In full-featured mode it provides a graphical user interface.
      settings: DeleteFcn=if exist('delete_tlblock','file')==2,delete_tlblock(gcbh);end  NameChangeFcn=if exist('rename_tlblock','file')==2,rename_tlblock(gcbh);end  OpenFcn=if exist('tl_open_blockdlg','file')==2,tl_open_blockdlg(gcbh);else,open_system(gcbh,'mask');end
      mask Help: eval('if exist(''tl_online_help'',''file'') == 2, tl_online_help(''Topic'',get_param(gcbh,''MaskType'')),end')
      mask Display: plot([0.5 0.5 4.5 4.5 0.5]/5,[2 4 4 2 2]/5,[0.5 1 1.5 2 2.5 3 3.5 4 4.3]/5,[2.1 2.7 2.4 3.9 3.0 3.2 2.05 2.8 3.1]/5,[1 1 1.3 1.3 1]/5,[1 1.3 1.3 1 1]/5,[3.7 3.7 4 4 3.7]/5,[1 1.3 1.3 1 1]/5);plot([-0.1, 1.05, NaN, -0.1, 1.05],[.01, .01, NaN, .99, .99]);
  Sqrt : Sqrt  SaturateOnIntegerOverflow=on  mask(TL_Sqrt){data={'date',730486}}
      settings: CopyFcn=if exist('tl_copyfcntllib', 'file') == 2, tl_copyfcntllib(gcbh); end;  DeleteFcn=if exist('delete_tlblock','file')==2,delete_tlblock(gcbh);end  NameChangeFcn=if exist('rename_tlblock','file')==2,rename_tlblock(gcbh);end  OpenFcn=if exist('tl_open_blockdlg','file')==2,tl_open_blockdlg(gcbh);else,open_system(gcbh,'parameter');end
      mask Help: eval(['if exist(''tl_online_help'',''file'') == 2, tl_online_help(''Topic'',''TL_Sqrt''),else, web([''jar:file:///'',matlabroot,''/help/toolbox/simulink/help.jar!/slref/' lower(get_param(gcbh,'Blocktype')) '.html''], ''-helpbrowser''),end'])
      mask Display: plot([-0.1, 1.05, NaN, -0.1, 1.05],[.01, .01, NaN, .99, .99]);
  Subsystem : Subsystem  Tag=TargetLink Simulation Frame  mask(TL_SimFrame){}
      mask help: TargetLink Simulation Frame
      settings: CopyFcn=if exist('tl_copyfcn','file'), tl_copyfcn(gcbh); end  NameChangeFcn=if exist('tl_framenamechangefcn','file'), tl_framenamechangefcn(gcbh); end
      settings: OpenFcn=|
      | if exist('open_tlsubsystem','file')==2
      |     open_tlsubsystem(gcbh);
      | else
      |        tlsubsystem = ...
      |            find_system(gcb, ...
      |            'LookUnderMasks','on', ...
      |            'FollowLinks','on', ...
      |            'Tag','MIL Subsystem');
      |        open_system(tlsubsystem);
      | end;
      mask Display: disp('TargetLink\nModel-\nin-the-loop\nmode')
  Sum : Sum  mask(TL_Sum){data={'date',730486}}
      settings: CopyFcn=if exist('tl_copyfcntllib', 'file') == 2, tl_copyfcntllib(gcbh); end;  DeleteFcn=if exist('delete_tlblock','file')==2,delete_tlblock(gcbh);end  NameChangeFcn=if exist('rename_tlblock','file')==2,rename_tlblock(gcbh);end  OpenFcn=if exist('tl_open_blockdlg','file')==2,tl_open_blockdlg(gcbh);else,open_system(gcbh,'parameter');end
      mask Help: eval(['if exist(''tl_online_help'',''file'') == 2, tl_online_help(''Topic'',''TL_Sum''),else, web([''jar:file:///'',matlabroot,''/help/toolbox/simulink/help.jar!/slref/' lower(get_param(gcbh,'Blocktype')) '.html''], ''-helpbrowser''),end'])
      mask Display: plot([-0.1, 1.05, NaN, -0.1, 1.05],[.01, .01, NaN, .99, .99]);
  Supported Simulink Blocks : Subsystem
      settings: OpenFcn=tl_openfcntllib('tllib_sl');
      mask Display: disp('Supported\nSimulink\nblocks')
  Switch : Switch  mask(TL_Switch){data={'date',730486}}
      settings: CopyFcn=if exist('tl_copyfcntllib', 'file') == 2, tl_copyfcntllib(gcbh); end;  DeleteFcn=if exist('delete_tlblock','file')==2,delete_tlblock(gcbh);end  NameChangeFcn=if exist('rename_tlblock','file')==2,rename_tlblock(gcbh);end  OpenFcn=if exist('tl_open_blockdlg','file')==2,tl_open_blockdlg(gcbh);else,open_system(gcbh,'parameter');end
      mask Help: eval(['if exist(''tl_online_help'',''file'') == 2, tl_online_help(''Topic'',''TL_Switch''),else, web([''jar:file:///'',matlabroot,''/help/toolbox/simulink/help.jar!/slref/' lower(get_param(gcbh,'Blocktype')) '.html''], ''-helpbrowser''),end'])
      mask Display: plot([-0.1, 1.05, NaN, -0.1, 1.05],[.01, .01, NaN, .99, .99]);
  TargetLink Main Dialog : Subsystem  mask(TL_MainDialog){data=[]}
      mask help: TargetLink Main Dialog block: In full-featured mode it provides the main graphical user interface to TargetLink.
      mask init: same as tllib/Addfile
      settings: CopyFcn=if exist('tl_copyfcn') == 2, tl_copyfcn(gcbh); end  OpenFcn=if exist('tl_open_blockdlg','file')==2,tl_open_blockdlg(gcbh);else,open_system(gcbh,'mask');end
      mask Help: eval('if exist(''tl_online_help'',''file'') == 2, tl_online_help(''Topic'',get_param(gcbh,''MaskType'')),end')
      mask Display: disp('TargetLink')
  Tool Selector : Subsystem  Description=Tool\nSelector  mask(TL_ToolSelector){data={'date',730486}}
      mask help: TargetLink Tool Selector block: In full-featured mode it can be used to start TargetLink tools.
      settings: DeleteFcn=if exist('tl_open_tool','file'),tl_open_tool('Delete',gcbh);end;  NameChangeFcn=if exist('rename_tlblock','file')==2,rename_tlblock(gcbh);end  OpenFcn=if exist('tl_open_tool','file')==2,tl_open_tool('Callback',gcbh);else open_system(gcbh,'mask');end
      mask Help: eval('if exist(''tl_online_help'',''file'') == 2, tl_online_help(''Topic'',get_param(gcbh,''MaskType'')),end')
      mask Display: disp(get_param(gcbh,'Description'));
  Trigonometric Function : Trigonometry  mask(TL_Trigonometry){data={'date',730486}}
      settings: CopyFcn=if exist('tl_copyfcntllib', 'file') == 2, tl_copyfcntllib(gcbh); end;  DeleteFcn=if exist('delete_tlblock','file')==2,delete_tlblock(gcbh);end  NameChangeFcn=if exist('rename_tlblock','file')==2,rename_tlblock(gcbh);end  OpenFcn=if exist('tl_open_blockdlg','file')==2,tl_open_blockdlg(gcbh);else,open_system(gcbh,'parameter');end
      mask Help: eval(['if exist(''tl_online_help'',''file'') == 2, tl_online_help(''Topic'',''TL_Trigonometry''),else, web([''jar:file:///'',matlabroot,''/help/toolbox/simulink/help.jar!/slref/' lower(get_param(gcbh,'Blocktype')) '.html''], ''-helpbrowser''),end'])
      mask Display: plot([-0.1, 1.05, NaN, -0.1, 1.05],[.01, .01, NaN, .99, .99]);
  Unit Delay : UnitDelay  SampleTime=-1  mask(TL_UnitDelay){data={'date',730486}}
      settings: CopyFcn=if exist('tl_copyfcntllib', 'file') == 2, tl_copyfcntllib(gcbh); end;  DeleteFcn=if exist('delete_tlblock','file')==2,delete_tlblock(gcbh);end  NameChangeFcn=if exist('rename_tlblock','file')==2,rename_tlblock(gcbh);end  OpenFcn=if exist('tl_open_blockdlg','file')==2,tl_open_blockdlg(gcbh);else,open_system(gcbh,'parameter');end
      mask Help: eval(['if exist(''tl_online_help'',''file'') == 2, tl_online_help(''Topic'',''TL_UnitDelay''),else, web([''jar:file:///'',matlabroot,''/help/toolbox/simulink/help.jar!/slref/' lower(get_param(gcbh,'Blocktype')) '.html''], ''-helpbrowser''),end'])
      mask Display: plot([-0.1, 1.05, NaN, -0.1, 1.05],[.01, .01, NaN, .99, .99]);
  Unit Delay Reset Enabled : Subsystem  mask(TL_UnitDelayRE){data={'date',730486}, dt=-1, X0=0, useexternaliv=on}
      mask prompts: dt "Sample time (-1 for inherited):"; X0 "Initial conditions:"; useexternaliv "Use external initial conditions"
      mask help: TargetLink Unit Delay Reset Enabled block: It is used to delay a signal by one sample step, according to reset options. In full-featured mode it provides a graphical user interface.
      settings: CopyFcn=if exist('tl_reset_reviewflag') == 2, tl_reset_reviewflag(gcbh); end;  DeleteFcn=if exist('delete_tlblock','file')==2,delete_tlblock(gcbh);end  NameChangeFcn=if exist('rename_tlblock','file')==2,rename_tlblock(gcbh);end  OpenFcn=if exist('tl_open_blockdlg','file')==2,tl_open_blockdlg(gcbh);else,open_system(gcbh,'mask');end
      mask Help: eval('if exist(''tl_online_help'',''file'') == 2, tl_online_help(''Topic'',get_param(gcbh,''MaskType'')),end')
      mask Display:
      | plot([-0.1, 1.05, NaN, -0.1, 1.05],[.01, .01, NaN, .99, .99]);
      | 
      | plot([.4 .6],[.5 .5]);
      | text(.5,.25,'z','HorizontalAlignment','center');
      | text(.5,.75,'1','HorizontalAlignment','center');
  dSPACE logo : Subsystem
      settings: OpenFcn=web('http://www.dspace.com/goto?targetlink', '-browser')
      mask Display: image(ds_get_icon('dspace_logo_bg_lightblue_m'))
  OutPort : Outport  mask(TL_Outport){data={'date',730486}}
      settings: CopyFcn=if exist('tl_copyfcntllib', 'file') == 2, tl_copyfcntllib(gcbh); end;  DeleteFcn=if exist('delete_tlblock','file')==2,delete_tlblock(gcbh);end  NameChangeFcn=if exist('rename_tlblock','file')==2,rename_tlblock(gcbh);end  OpenFcn=if exist('tl_open_blockdlg','file')==2,tl_open_blockdlg(gcbh);else,open_system(gcbh,'parameter');end
      mask Help: eval(['if exist(''tl_online_help'',''file'') == 2, tl_online_help(''Topic'',''TL_Outport''),else, web([''jar:file:///'',matlabroot,''/help/toolbox/simulink/help.jar!/slref/' lower(get_param(gcbh,'Blocktype')) '.html''], ''-helpbrowser''),end'])
      mask Display: plot([0.2 0.35 NaN 0.65 0.8],[0 1 NaN 0 1]);
  Bus Outport : Outport  Port=2  mask(TL_BusOutport){data={'date',730486}}
      settings: CopyFcn=if exist('tl_copyfcntllib', 'file') == 2, tl_copyfcntllib(gcbh); end;  DeleteFcn=if exist('delete_tlblock','file')==2,delete_tlblock(gcbh);end  NameChangeFcn=if exist('rename_tlblock','file')==2,rename_tlblock(gcbh);end  OpenFcn=if exist('tl_open_blockdlg','file')==2,tl_open_blockdlg(gcbh);else,open_system(gcbh,'parameter');end
      mask Help: eval(['if exist(''tl_online_help'',''file'') == 2, tl_online_help(''Topic'',''TL_Outport''),else, web([''jar:file:///'',matlabroot,''/help/toolbox/simulink/help.jar!/slref/' lower(get_param(gcbh,'Blocktype')) '.html''], ''-helpbrowser''),end'])
      mask Display: plot([0.2 0.35 NaN 0.65 0.8],[0 1 NaN 0 1]);
